simulink model "sl_subsys_iferr1"  (Simulink 7.6)
settings: Solver=FixedStepDiscrete  StartTime=0.0  StopTime=10.0  FixedStep=1  RelTol=1e-3
Description:
  | Invalid If block and action subsystem
  | 
  | The following model is an example of an if-action block erroneously executing the
  | action subsystem 'If body'. Block B is driving the 'If body' block and
  | must execute before the 'If' block. However, the 'If body' block needs to execute
  | before 'B'. This poses a causality problem.  To execute 'If body', we must
  | first execute 'If', before 'B'. However, 'B' must execute prior to
  | "If' and, hence, the error.
settings Model: Creator=The MathWorks Inc.  CovMetricSettings=d  ExtModeAutoUpdateStatusClock=off
settings OptimizationCC: BlockReduction=off  BooleanDataType=off  InlineInvariantSignals=on  InitFltsAndDblsToZero=on
settings DebuggingCC: SaveWithParameterizedLinksMsg=none  SignalResolutionControl=TryResolveAllWithWarning  SolverPrmCheckMsg=none  MultiTaskDSMMsg=warning  MultiTaskCondExecSysMsg=none
settings HardwareCC: TargetUnknown=on
settings RTWCC: IncludeERTFirstTime=on
settings CodeAppCC: CustomSymbolStrFcn=$F$N$M
settings GRTTargetCC: TargetFcnLib=ansi_tfl_tmw.mat

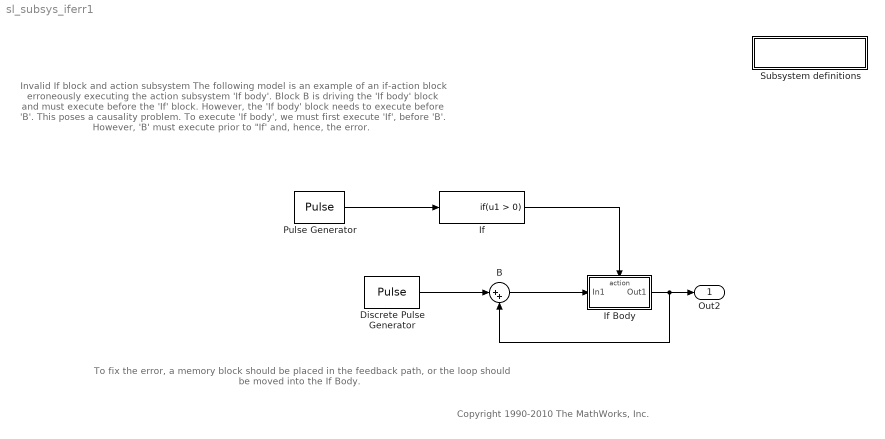
== system sl_subsys_iferr1 ==
  note: Invalid If block and action subsystem
      |
      | The following model is an example of an if-action block erroneously executing the
      | action subsystem 'If body'. Block B is driving the 'If body' block and
      | must execute before the 'If' block. However, the 'If body' block needs to execute
      | before 'B'. This poses a causality problem.  To execute 'If body', we must
      | first execute 'If', before 'B'. However, 'B' must execute prior to
      | "If' and, hence, the error.
  note: To fix the error, a memory block should be placed in the feedback path, or
      | the loop should be moved into the If Body.
  note: Copyright 1990-2010 The MathWorks, Inc.
  " Subsystem definitions" : Subsystem
      settings: OpenFcn=helpview([matlabroot,'/toolbox/simulink/simdemos/simfeatures/html/sl_subsys_definitions.html']);
      mask Display: disp('Subsystem\ndefinitions')
  B : Sum  Inputs=|++  SaturateOnIntegerOverflow=on  InputSameDT=on  OutDataTypeStr=Inherit: Same as first input
  Discrete Pulse Generator : DiscretePulseGenerator
  If : If  ShowElse=off
  If Body : Subsystem  TreatAsAtomicUnit=on
  Pulse Generator : DiscretePulseGenerator
  Out2 : Outport
  wires:
  If/1 -> If Body/Action
  Pulse Generator/1 -> If/1
  Discrete Pulse Generator/1 -> B/1
  If Body/1(Out1) -> Out2/1, B/2
  B/1 -> If Body/1(In1)

== system sl_subsys_iferr1/ Subsystem definitions ==

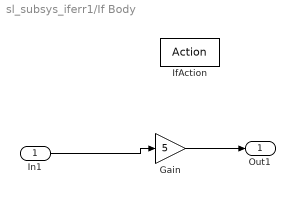
== system sl_subsys_iferr1/If Body ==
  In1 : Inport
  IfAction : ActionPort  ActionType=then
  Gain : Gain  Gain=5  SaturateOnIntegerOverflow=on  OutDataTypeStr=Inherit: Same as input  ParamDataTypeStr=Inherit: Same as input
  Out1 : Outport
  wires:
  In1/1 -> Gain/1
  Gain/1 -> Out1/1
